simulink subsystem "PvtSubSys_VSM_ALL"  (R2020b)
settings: Solver=VariableStepAuto  StartTime=0.0  StopTime=10.0  RelTol=1e-3
values from neighbouring files (symbols this model uses):
  P_VSM_NOH_Act_Req = 0    [VSM_All.sldd]
  P_VSM_NOH_Swt_Req = 0    [VSM_All.sldd]
undefined symbols (not defined in the file or in its folder): ACC_STATE, HWA_STATE, LCK_STATE, P_VSM_ACCSOS_SW, P_VSM_AESSwtReq, P_VSM_CruiseFunUserInputMappingWays, P_VSM_ELKSwtReq, P_VSM_ESS_VehSwtReq, P_VSM_HWA_DMS_Enable, P_VSM_ICA_HandsOffSwtReq, P_VSM_IntelligentEvaSwtReq, P_VSM_ISLSwtReq, P_VSM_LCKSwtReq, P_VSM_LDWSwtReq, P_VSM_LKASwtReq, P_VSM_LSSSwtReq, P_VSM_PowerTrainConfig, P_VSM_SOSContinueTime, P_VSM_SOSSpdLimit, P_VSM_TSR_Dis_keep_SPL_Table, P_VSM_TSR_Dis_keep_SPLend, P_VSM_TSR_Dis_keep_TS_Table, P_VSM_TSR_Ena_SPLSupp_Table, P_VSM_TSR_Ena_TS_Table, P_VSM_TSR_SLIF_Speed_High, P_VSM_TSR_SLIF_Speed_Low, P_VSM_TSR_SLW_SnvtySwitch, P_VSM_TSR_SLW_Speed_Delta_disable, P_VSM_TSR_SLW_Speed_Delta_enable, P_VSM_TSR_SLW_Speed_High, P_VSM_TSR_SLW_Speed_Low, P_VSM_TSR_SLW_TrafEyeAvtiveDist, P_VSM_TSR_SLW_Warning_Time, P_VSM_TSR_SteerWheelAngle, P_VSM_TSR_SWS_speed_withDir, P_VSM_TSR_SWS_speed_woDir, P_VSM_TSRSwtReq, P_VSM_TSRWarnSwtReq, TJA_STATE, User_LC_ALCswt, User_LC_DrvConfirm, User_LC_DrvLCswt, User_LC_DrvOverride, User_LC_LeTurnNextLineReq, User_LC_RiTurnNextLineReq, User_LC_TurnMostLeLineReq, User_LC_TurnMostRiLineReq, User_LeTurnLmpOn, User_RiTurnLmpOn
libraries: simulink x51
(part 7 of 7)

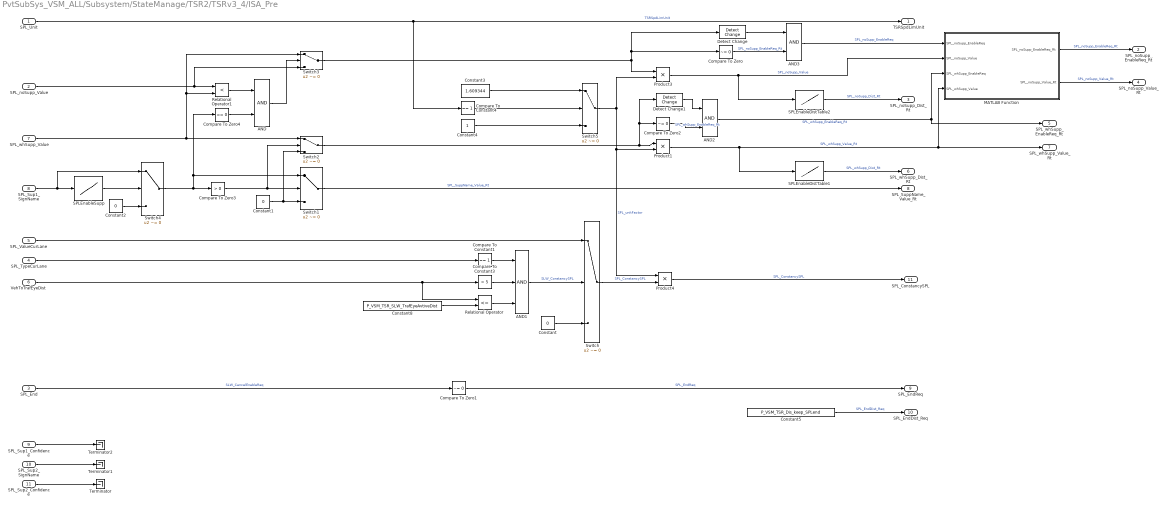
== system PvtSubSys_VSM_ALL/Subsystem/StateManage/TSR2/TSRv3_4/ISA_Pre ==
  SPL_Unit : Inport  OutDataTypeStr=uint8
  SPL_noSupp_Value : Inport  Port=2  OutDataTypeStr=uint8
  SPL_End : Inport  Port=3  OutDataTypeStr=uint8
  SPL_TypeCurLane : Inport  Port=4  OutDataTypeStr=uint8
  SPL_ValueCurLane : Inport  Port=5  OutDataTypeStr=uint8
  VehToTrafEyeDist : Inport  Port=6  OutDataTypeStr=uint16
  SPL_whSupp_Value : Inport  Port=7
  SPL_Sup1_SignName : Inport  Port=8  OutDataTypeStr=uint8
  SPL_Sup1_Confidence : Inport  Port=9  OutDataTypeStr=single
  SPL_Sup2_SignName : Inport  Port=10  OutDataTypeStr=uint8
  SPL_Sup2_Confidence : Inport  Port=11  OutDataTypeStr=single
  AND : Logic  AllPortsSameDT=off  OutDataTypeStr=boolean
  AND1 : Logic  Inputs=3  AllPortsSameDT=off  OutDataTypeStr=boolean
  AND2 : Logic  AllPortsSameDT=off  OutDataTypeStr=boolean
  AND3 : Logic  AllPortsSameDT=off  OutDataTypeStr=boolean
  Compare To Constant1 : simulink/Logic and Bit Operations/Compare To Constant  relop===  const=1  OutDataTypeStr=boolean
  Compare To Constant3 : simulink/Logic and Bit Operations/Compare To Constant  relop=>  const=5  OutDataTypeStr=boolean
  Compare To Constant4 : simulink/Logic and Bit Operations/Compare To Constant  relop===  const=1  OutDataTypeStr=boolean
  Compare To Zero : simulink/Logic and Bit Operations/Compare To Zero  relop=~=  OutDataTypeStr=boolean
  Compare To Zero1 : simulink/Logic and Bit Operations/Compare To Zero  relop=~=  OutDataTypeStr=boolean
  Compare To Zero2 : simulink/Logic and Bit Operations/Compare To Zero  relop=~=  OutDataTypeStr=boolean
  Compare To Zero3 : simulink/Logic and Bit Operations/Compare To Zero  relop=>  OutDataTypeStr=boolean
  Compare To Zero4 : simulink/Logic and Bit Operations/Compare To Zero  relop===  OutDataTypeStr=boolean
  Constant : Constant  Value=0  OutDataTypeStr=uint8
  Constant1 : Constant  Value=0  OutDataTypeStr=Inherit: Inherit via back propagation
  Constant2 : Constant  Value=0  OutDataTypeStr=Inherit: Inherit via back propagation
  Constant3 : Constant  Value=1.609344
  Constant4 : Constant
  Constant5 : Constant  Value=P_VSM_TSR_Dis_keep_SPLend  OutDataTypeStr=single
  Constant8 : Constant  Value=P_VSM_TSR_SLW_TrafEyeAvtiveDist
  Detect Change : simulink/Logic and Bit Operations/Detect Change  vinit=0  OutDataTypeStr=boolean
  Detect Change1 : simulink/Logic and Bit Operations/Detect Change  vinit=0  OutDataTypeStr=boolean
  MATLAB Function : MATLAB Function  TreatAsAtomicUnit=on
  Product1 : Product  OutDataTypeStr=uint8
  Product3 : Product  OutDataTypeStr=uint8
  Product4 : Product  OutDataTypeStr=uint8
  Relational Operator : RelationalOperator  Operator=<=  OutDataTypeStr=boolean  RndMeth=Simplest
  Relational Operator1 : RelationalOperator  Operator=<  OutDataTypeStr=boolean  RndMeth=Simplest
  SPLEnableDistTable1 : Lookup_n-D  NumberOfTableDimensions=1  BreakpointsForDimension1=[0:10:150]  BreakpointsForDimension1DataTypeStr=uint8  Table=P_VSM_TSR_Dis_keep_SPL_Table  TableDataTypeStr=Inherit: Inherit from 'Table data'  InterpMethod=Flat  ExtrapMethod=Cubic spline  InternalRulePriority=Speed  OutDataTypeStr=single  RndMeth=Simplest  InputSameDT=on
  SPLEnableDistTable2 : Lookup_n-D  NumberOfTableDimensions=1  BreakpointsForDimension1=[0:10:150]  BreakpointsForDimension1DataTypeStr=uint8  Table=P_VSM_TSR_Dis_keep_SPL_Table  TableDataTypeStr=Inherit: Inherit from 'Table data'  InterpMethod=Flat  ExtrapMethod=Cubic spline  InternalRulePriority=Speed  OutDataTypeStr=single  RndMeth=Simplest  InputSameDT=on
  SPLEnableSupp : Lookup_n-D  NumberOfTableDimensions=1  BreakpointsForDimension1=[0:1:0x16]  BreakpointsForDimension1DataTypeStr=uint8  Table=P_VSM_TSR_Ena_SPLSupp_Table  TableDataTypeStr=Inherit: Inherit from 'Table data'  InterpMethod=Flat  ExtrapMethod=Cubic spline  InternalRulePriority=Speed  OutDataTypeStr=Inherit: Inherit via back propagation  RndMeth=Simplest  InputSameDT=on
  Switch : Switch  Criteria=u2 ~= 0  OutDataTypeStr=uint8
  Switch{1..4} (4 alike) : Switch  Criteria=u2 ~= 0
  Switch5 : Switch  Criteria=u2 ~= 0  Threshold=1  OutDataTypeStr=single
  Terminator : Terminator
  Terminator1 : Terminator
  Terminator2 : Terminator
  TSRSpdLimUnit : Outport  OutDataTypeStr=uint8
  SPL_noSupp_EnableReq_Rt : Outport  Port=2  OutDataTypeStr=boolean
  SPL_noSupp_Dist_Rt : Outport  Port=3  OutDataTypeStr=single
  SPL_noSupp_Value_Rt : Outport  Port=4  OutDataTypeStr=uint8
  SPL_whSupp_EnableReq_Rt : Outport  Port=5  OutDataTypeStr=boolean
  SPL_whSupp_Dist_Rt : Outport  Port=6  OutDataTypeStr=single
  SPL_whSupp_Value_Rt : Outport  Port=7  OutDataTypeStr=uint8
  SPL_SuppName_Value_Rt : Outport  Port=8
  SPL_EndReq : Outport  Port=9  OutDataTypeStr=boolean
  SPL_EndDist_Req : Outport  Port=10  OutDataTypeStr=single
  SPL_ConstancySPL : Outport  Port=11  OutDataTypeStr=uint8
  wires:
  Compare To Zero1/1 -> SPL_EndReq/1  "SPL_EndReq"
  Switch3/1 -> Detect Change/1, Compare To Zero/1, Product3/1
  AND3/1 -> MATLAB Function/1(SPL_noSupp_EnableReq)  "SPL_noSupp_EnableReq"
  Compare To Constant3/1 -> AND1/2
  AND1/1 -> Switch/2  "SLW_ConstancySPL"
  SPL_ValueCurLane/1 -> Switch/1
  SPL_TypeCurLane/1 -> Compare To Constant1/1
  Product3/1 -> MATLAB Function/2(SPL_noSupp_Value), SPLEnableDistTable2/1  "SPL_noSupp_Value"
  Relational Operator/1 -> AND1/3
  Constant8/1 -> Relational Operator/2
  SPLEnableDistTable2/1 -> SPL_noSupp_Dist_Rt/1  "SPL_noSupp_Dist_Rt"
  Constant5/1 -> SPL_EndDist_Req/1  "SPL_EndDist_Req"
  SPL_End/1 -> Compare To Zero1/1  "SLW_CancelEnableReq"
  VehToTrafEyeDist/1 -> Relational Operator/1, Compare To Constant3/1
  Compare To Constant1/1 -> AND1/1
  Switch4/1 -> Compare To Zero4/1, Switch1/1, Compare To Zero3/1
  SPLEnableDistTable1/1 -> SPL_whSupp_Dist_Rt/1  "SPL_whSupp_Dist_Rt"
  SPL_Sup2_Confidence/1 -> Terminator/1
  SPL_Sup1_Confidence/1 -> Terminator2/1
  SPL_Sup2_SignName/1 -> Terminator1/1
  Switch2/1 -> Detect Change1/1, Compare To Zero2/1, Product1/1
  Product1/1 -> SPLEnableDistTable1/1, SPL_whSupp_Value_Rt/1, MATLAB Function/4(SPL_whSupp_Value)  "SPL_whSupp_Value_Rt"
  AND2/1 -> SPL_whSupp_EnableReq_Rt/1, MATLAB Function/3(SPL_whSupp_EnableReq)  "SPL_whSupp_EnableReq_Rt"
  Compare To Constant4/1 -> Switch5/2
  SPL_Unit/1 -> Compare To Constant4/1, TSRSpdLimUnit/1  "TSRSpdLimUnit"
  Constant3/1 -> Switch5/1
  Constant4/1 -> Switch5/3
  Switch5/1 -> Product1/2, Product4/1, Product3/2  "SPL_unitFactor"
  Constant/1 -> Switch/3
  Switch/1 -> Product4/2  "SPL_ConstancySPL"
  Product4/1 -> SPL_ConstancySPL/1  "SPL_ConstancySPL"
  Compare To Zero3/1 -> Switch2/2, Switch1/2
  SPL_whSupp_Value/1 -> Switch2/1, Switch3/1, Relational Operator1/2
  Switch1/1 -> SPL_SuppName_Value_Rt/1  "SPL_SuppName_Value_Rt"
  Constant1/1 -> Switch2/3, Switch1/3
  SPL_noSupp_Value/1 -> Switch3/3, Relational Operator1/1
  Relational Operator1/1 -> AND/1
  Compare To Zero4/1 -> AND/2
  AND/1 -> Switch3/2
  SPL_Sup1_SignName/1 -> Switch4/1, SPLEnableSupp/1
  SPLEnableSupp/1 -> Switch4/2
  Constant2/1 -> Switch4/3
  Detect Change/1 -> AND3/1
  Compare To Zero/1 -> AND3/2  "SPL_noSupp_EnableReq_Rt"
  MATLAB Function/2(SPL_noSupp_Value_Rt) -> SPL_noSupp_Value_Rt/1  "SPL_noSupp_Value_Rt"
  MATLAB Function/1(SPL_noSupp_EnableReq_Rt) -> SPL_noSupp_EnableReq_Rt/1  "SPL_noSupp_EnableReq_Rt"
  Detect Change1/1 -> AND2/1
  Compare To Zero2/1 -> AND2/2  "SPL_whSupp_EnableReq_Rt"

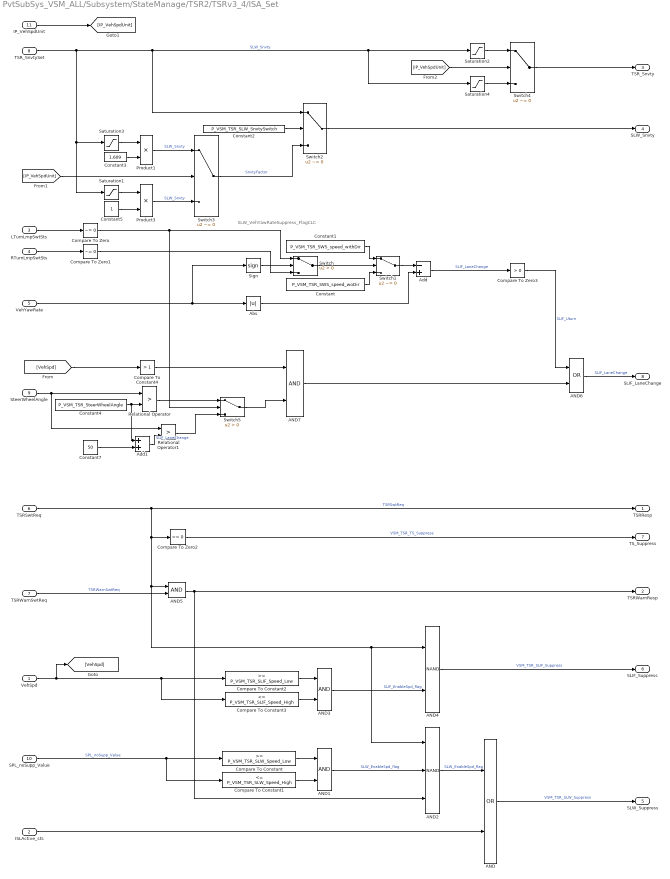
== system PvtSubSys_VSM_ALL/Subsystem/StateManage/TSR2/TSRv3_4/ISA_Set ==
  note: SLW_VehYawRateSuppress_FlagCLC
  VehSpd : Inport  OutDataTypeStr=single
  ISLActive_sts : Inport  Port=2  OutDataTypeStr=boolean
  LTurnLmpSwtSts : Inport  Port=3  OutDataTypeStr=boolean
  RTurnLmpSwtSts : Inport  Port=4  OutDataTypeStr=boolean
  VehYawRate : Inport  Port=5  OutDataTypeStr=single
  TSRSwtReq : Inport  Port=6
  TSRWarnSwtReq : Inport  Port=7
  TSR_SnvtySet : Inport  Port=8
  SteerWheelAngle : Inport  Port=9  OutDataTypeStr=single
  SPL_noSupp_Value : Inport  Port=10  OutDataTypeStr=uint8
  IP_VehSpdUnit : Inport  Port=11  OutDataTypeStr=boolean
  AND : Logic  Operator=OR  AllPortsSameDT=off  OutDataTypeStr=boolean
  AND{1,3,5,7} (4 alike) : Logic  AllPortsSameDT=off  OutDataTypeStr=boolean
  AND2 : Logic  Operator=NAND  Inputs=3  AllPortsSameDT=off  OutDataTypeStr=boolean
  AND4 : Logic  Operator=NAND  AllPortsSameDT=off  OutDataTypeStr=boolean
  AND6 : Logic  Operator=OR  AllPortsSameDT=off  OutDataTypeStr=boolean
  Abs : Abs
  Add : Sum  Inputs=-+
  Add1 : Sum
  Compare To Constant : simulink/Logic and Bit Operations/Compare To Constant  relop=>=  const=P_VSM_TSR_SLW_Speed_Low  OutDataTypeStr=boolean
  Compare To Constant1 : simulink/Logic and Bit Operations/Compare To Constant  relop=<=  const=P_VSM_TSR_SLW_Speed_High  OutDataTypeStr=boolean
  Compare To Constant2 : simulink/Logic and Bit Operations/Compare To Constant  relop=>=  const=P_VSM_TSR_SLIF_Speed_Low  OutDataTypeStr=boolean
  Compare To Constant3 : simulink/Logic and Bit Operations/Compare To Constant  relop=<=  const=P_VSM_TSR_SLIF_Speed_High  OutDataTypeStr=boolean
  Compare To Constant4 : simulink/Logic and Bit Operations/Compare To Constant  relop=>  const=1  OutDataTypeStr=boolean
  Compare To Zero : simulink/Logic and Bit Operations/Compare To Zero  relop=~=  OutDataTypeStr=boolean
  Compare To Zero1 : simulink/Logic and Bit Operations/Compare To Zero  relop=~=  OutDataTypeStr=boolean
  Compare To Zero2 : simulink/Logic and Bit Operations/Compare To Zero  relop===  OutDataTypeStr=boolean
  Compare To Zero3 : simulink/Logic and Bit Operations/Compare To Zero  relop=>  OutDataTypeStr=uint8
  Constant : Constant  Value=P_VSM_TSR_SWS_speed_woDir
  Constant1 : Constant  Value=P_VSM_TSR_SWS_speed_withDir
  Constant2 : Constant  Value=P_VSM_TSR_SLW_SnvtySwitch
  Constant3 : Constant  Value=1.609  OutDataTypeStr=single
  Constant4 : Constant  Value=P_VSM_TSR_SteerWheelAngle
  Constant5 : Constant  OutDataTypeStr=Inherit: Inherit via back propagation
  Constant7 : Constant  Value=50
  Product1 : Product  OutDataTypeStr=single
  Product3 : Product  OutDataTypeStr=single
  Relational Operator : RelationalOperator  Operator=>  OutDataTypeStr=boolean  RndMeth=Simplest
  Relational Operator1 : RelationalOperator  Operator=>  OutDataTypeStr=boolean  RndMeth=Simplest
  Saturation1 : Saturate  UpperLimit=10  LowerLimit=-10
  Saturation2 : Saturate  UpperLimit=5  LowerLimit=-5
  Saturation3 : Saturate  UpperLimit=5  LowerLimit=-5
  Saturation4 : Saturate  UpperLimit=10  LowerLimit=-10
  Sign : Signum
  Switch : Switch  Criteria=u2 > Threshold
  Switch1 : Switch  Criteria=u2 ~= 0
  Switch2 : Switch  Criteria=u2 ~= 0  OutDataTypeStr=single
  Switch3 : Switch  Criteria=u2 ~= 0  Threshold=1  OutDataTypeStr=single
  Switch4 : Switch  Criteria=u2 ~= 0  OutDataTypeStr=int8
  Switch5 : Switch  Criteria=u2 > Threshold
  TSRResp : Outport
  TSRWarnResp : Outport  Port=2
  TSR_Snvty : Outport  Port=3  OutDataTypeStr=int8
  SLW_Snvty : Outport  Port=4  OutDataTypeStr=single
  SLW_Suppress : Outport  Port=5
  SLIF_Suppress : Outport  Port=6
  TS_Suppress : Outport  Port=7
  SLIF_LaneChange : Outport  Port=8  OutDataTypeStr=boolean
  wires:
  AND4/1 -> SLIF_Suppress/1  "VSM_TSR_SLIF_Suppress"
  Abs/1 -> Add/2
  VehYawRate/1 -> Abs/1, Sign/1
  Sign/1 -> Switch/2
  Compare To Zero/1 -> Switch/1, Switch5/2
  RTurnLmpSwtSts/1 -> Compare To Zero1/1
  Switch1/1 -> Add/1
  Compare To Zero1/1 -> Switch/3
  Constant/1 -> Switch1/3
  Switch/1 -> Switch1/2
  Constant1/1 -> Switch1/1
  LTurnLmpSwtSts/1 -> Compare To Zero/1
  Add/1 -> Compare To Zero3/1  "SLIF_LaneChange"
  AND/1 -> SLW_Suppress/1  "VSM_TSR_SLW_Suppress"
  ISLActive_sts/1 -> AND/2
  Compare To Constant1/1 -> AND1/2
  Compare To Constant/1 -> AND1/1
  AND1/1 -> AND2/2  "SLW_EnableSpd_flag"
  AND5/1 -> AND2/3, TSRWarnResp/1
  AND2/1 -> AND/1  "SLW_EnableSpd_flag"
  Compare To Constant2/1 -> AND3/1
  AND3/1 -> AND4/2  "SLIF_EnableSpd_flag"
  Compare To Constant3/1 -> AND3/2
  VehSpd/1 -> [VehSpd], Compare To Constant3/1, Compare To Constant2/1
  TSRSwtReq/1 -> Compare To Zero2/1, AND2/1, AND4/1, AND5/1, TSRResp/1  "TSRSwtReq"
  TSRWarnSwtReq/1 -> AND5/2  "TSRWarnSwtReq"
  Compare To Zero2/1 -> TS_Suppress/1  "VSM_TSR_TS_Suppress"
  Compare To Zero3/1 -> AND6/1  "SLIF_Uturn"
  Constant2/1 -> Switch2/2
  Switch2/1 -> SLW_Snvty/1
  SteerWheelAngle/1 -> Relational Operator1/1, Relational Operator/1
  Constant4/1 -> Add1/1, Relational Operator/2
  Switch5/1 -> AND7/2
  AND6/1 -> SLIF_LaneChange/1  "SLIF_LaneChange"
  [VehSpd] -> Compare To Constant4/1
  Compare To Constant4/1 -> AND7/1
  AND7/1 -> AND6/2
  SPL_noSupp_Value/1 -> Compare To Constant1/1, Compare To Constant/1  "SPL_noSupp_Value"
  Switch3/1 -> Switch2/3  "SnvtyFactor"
  [IP_VehSpdUnit] -> Switch3/2
  Constant5/1 -> Product3/2
  TSR_SnvtySet/1 -> Saturation1/1, Saturation3/1, Switch2/1, Saturation4/1, Saturation2/1  "SLW_Snvty"
  Constant3/1 -> Product1/2
  Product1/1 -> Switch3/1  "SLW_Snvty"
  Product3/1 -> Switch3/3  "SLW_Snvty"
  Saturation3/1 -> Product1/1
  Saturation1/1 -> Product3/1
  Switch4/1 -> TSR_Snvty/1
  IP_VehSpdUnit/1 -> [IP_VehSpdUnit]
  [IP_VehSpdUnit] -> Switch4/2
  Saturation2/1 -> Switch4/1
  Saturation4/1 -> Switch4/3
  Relational Operator/1 -> Switch5/1
  Constant7/1 -> Add1/2
  Add1/1 -> Relational Operator1/2  "SLIF_LaneChange"
  Relational Operator1/1 -> Switch5/3

== system PvtSubSys_VSM_ALL/Subsystem/StateManage/TSR2/TSRv3_4/ISAnoSupp ==
  SLW_Snvty : Inport  OutDataTypeStr=single
  SLIF_VehSpdValue : Inport  Port=2  OutDataTypeStr=single
  SLIF_LaneChange : Inport  Port=3  OutDataTypeStr=boolean
  SLIF_Suppress : Inport  Port=4  OutDataTypeStr=boolean
  SLW_Suppress : Inport  Port=5
  SPL_noSupp_EnableReq : Inport  Port=6  OutDataTypeStr=boolean
  SPL_noSupp_Dist_Req : Inport  Port=7  OutDataTypeStr=single
  SPL_noSupp_Value_Req : Inport  Port=8  OutDataTypeStr=uint8
  SPL_End_Req : Inport  Port=9  OutDataTypeStr=boolean
  SPL_EndDist_Req : Inport  Port=10  OutDataTypeStr=single
  SPL_Constancy_Req : Inport  Port=11  OutDataTypeStr=uint8
  Chart1 : Stateflow chart  TreatAsAtomicUnit=on
  Constant : Constant  Value=0  OutDataTypeStr=Inherit: Inherit via back propagation
  Constant1 : Constant  Value=P_VSM_TSR_SLW_Speed_Delta_enable
  Constant13 : Constant  Value=P_VSM_TSR_SLW_Warning_Time
  Constant2 : Constant  Value=P_VSM_TSR_SLW_SnvtySwitch
  Constant3 : Constant  Value=P_VSM_TSR_SLW_Speed_Delta_disable
  Ground : Ground
  Switch{,1..3} (4 alike) : Switch  Criteria=u2 ~= 0
  Switch4 : Switch  Criteria=u2 ~= 0  OutDataTypeStr=single
  Terminator : Terminator
  Terminator1 : Terminator
  Unit Delay : UnitDelay  SampleTime=-1  HasFrameUpgradeWarning=on
  TSRSpdLimWarn : Outport
  TSRSpdLimCfdc : Outport  Port=2  OutDataTypeStr=uint8
  TSRSpdLim : Outport  Port=3
  TSRSpdLimSts : Outport  Port=4
  SLW_Enable : Outport  Port=5
  SLW_SpdLimValue : Outport  Port=6  OutDataTypeStr=uint8
  SPL_noSupp_Dist_Remain : Outport  Port=7  OutDataTypeStr=single
  SPLnoSuppDistKeep : Outport  Port=8
  SPL_noSupp_Value_Remain : Outport  Port=9
  wires:
  SLIF_Suppress/1 -> Switch/2, Switch1/2, Switch2/2  "SLIF_Suppress"
  SLIF_VehSpdValue/1 -> Chart1/1(SLIF_VehSpdValue)
  Chart1/4(TSRSpdLimWarn) -> SLW_Enable/1, Switch3/3  "SLW_Enable"
  Chart1/8(SLIF_SpdLimValue) -> Unit Delay/1, SPL_noSupp_Value_Remain/1  "SPL_noSupp_Value_Remain"
  Chart1/3(SLIF_SpdLimCoded) -> Switch2/3
  Chart1/6(SLIF_EnableDist) -> SPLnoSuppDistKeep/1  "SPLdistKeep"
  Chart1/7(SLIF_RemainDist) -> SPL_noSupp_Dist_Remain/1  "SPL_noSupp_Dist_Remain"
  Chart1/1(TSRSpdLimSts) -> Switch/3
  Chart1/9(SLW_SpdLimValue) -> SLW_SpdLimValue/1  "SLW_SpdLimValue"
  Chart1/2(TSRSpdLimCfdc) -> Switch1/3
  Switch/1 -> TSRSpdLimSts/1  "TSRSpdLimSts"
  Switch1/1 -> TSRSpdLimCfdc/1  "TSRSpdLimCfdc"
  Switch2/1 -> TSRSpdLim/1  "TSRSpdLim"
  Switch3/1 -> TSRSpdLimWarn/1  "TSRSpdLimWarn"
  SLW_Suppress/1 -> Switch3/2
  Constant/1 -> Switch3/1, Switch2/1, Switch1/1, Switch/1
  Constant1/1 -> Chart1/10(APV_SLW_Speed_Delta_enable)
  Constant3/1 -> Chart1/11(APV_SLW_Speed_Delta_disable)
  Constant13/1 -> Chart1/12(APV_SLW_Warning_Time)
  SPL_noSupp_EnableReq/1 -> Chart1/3(SLIF_EnableReq)  "VSM_TSR_SPL_noSupp_EnableReq"
  SPL_noSupp_Dist_Req/1 -> Chart1/4(SLIF_EnableDistReq)  "VSM_TSR_SPL_noSupp_Dist_Req"
  SPL_noSupp_Value_Req/1 -> Chart1/5(SLIF_SpdLimValueReq)  "VSM_TSR_SPL_noSupp_Value_Req"
  SPL_Constancy_Req/1 -> Chart1/6(SLIF_ConstancySPL)  "VSM_TSR_SPL_Constancy_Req"
  SPL_End_Req/1 -> Chart1/7(SLIF_End_Req)  "VSM_TSR_SPL_End_Req"
  SPL_EndDist_Req/1 -> Chart1/8(SLIF_EndDist_Req)  "VSM_TSR_SPL_EndDist_Req"
  SLIF_LaneChange/1 -> Chart1/9(SLIF_Disable)
  Ground/1 -> Chart1/13(SPL_SuppName_Value_Req)
  Chart1/10(SPL_SuppName) -> Terminator/1
  Constant2/1 -> Switch4/2
  SLW_Snvty/1 -> Switch4/3  "SLW_Snvty"
  Switch4/1 -> Chart1/2(SLW_Snvty)
  Unit Delay/1 -> Switch4/1
  Chart1/5(SLIF_Enable) -> Terminator1/1  "SLW_Enable"

== system PvtSubSys_VSM_ALL/Subsystem/StateManage/TSR2/TSRv3_4/ISAwhSupp ==
  SLW_Snvty : Inport  OutDataTypeStr=single
  SLIF_VehSpdValue : Inport  Port=2
  SLIF_LaneChange : Inport  Port=3  OutDataTypeStr=boolean
  SLIF_Suppress : Inport  Port=4  OutDataTypeStr=boolean
  SLW_Suppress : Inport  Port=5
  SPL_whSupp_EnableReq : Inport  Port=6  OutDataTypeStr=boolean
  SPL_whSupp_Dist_Req : Inport  Port=7  OutDataTypeStr=single
  SPL_whSupp_Value_Req : Inport  Port=8  OutDataTypeStr=uint8
  SPL_SuppName_Value_Req : Inport  Port=9  OutDataTypeStr=uint8
  SPL_End_Req : Inport  Port=10  OutDataTypeStr=boolean
  SPL_EndDist_Req : Inport  Port=11  OutDataTypeStr=single
  SPL_Constancy_Req : Inport  Port=12  OutDataTypeStr=uint8
  Chart1 : Stateflow chart  TreatAsAtomicUnit=on
  Constant : Constant  Value=0  OutDataTypeStr=Inherit: Inherit via back propagation
  Constant1 : Constant  Value=P_VSM_TSR_SLW_Speed_Delta_enable
  Constant13 : Constant  Value=P_VSM_TSR_SLW_Warning_Time
  Constant2 : Constant  Value=P_VSM_TSR_SLW_SnvtySwitch
  Constant3 : Constant  Value=P_VSM_TSR_SLW_Speed_Delta_disable
  Switch2 : Switch  Criteria=u2 ~= 0
  Switch3 : Switch  Criteria=u2 ~= 0
  Switch4 : Switch  Criteria=u2 ~= 0  OutDataTypeStr=single
  Terminator{,1,3..4} (4 alike) : Terminator
  Unit Delay : UnitDelay  SampleTime=-1  HasFrameUpgradeWarning=on
  TSRConSpdLimWarn : Outport
  TSRConSpdLim : Outport  Port=2
  SPL_whSupp_Dist_Remain : Outport  Port=3  OutDataTypeStr=single
  SPL_whSupp_Value_Remain : Outport  Port=4  OutDataTypeStr=uint8
  SPL_SuppName_Value_Remain : Outport  Port=5  OutDataTypeStr=uint8
  SPLwhSuppDistKeep : Outport  Port=6  OutDataTypeStr=single
  wires:
  Constant/1 -> Switch2/1, Switch3/1
  Chart1/2(TSRSpdLimCfdc) -> Terminator1/1
  Chart1/1(TSRSpdLimSts) -> Terminator/1
  SLW_Suppress/1 -> Switch3/2
  Chart1/4(TSRSpdLimWarn) -> Switch3/3
  Switch2/1 -> TSRConSpdLim/1  "TSRConSpdLim"
  Chart1/3(SLIF_SpdLimCoded) -> Switch2/3
  SPL_EndDist_Req/1 -> Chart1/8(SLIF_EndDist_Req)
  Chart1/6(SLIF_EnableDist) -> SPLwhSuppDistKeep/1  "SPLwhSuppDistKeep"
  Switch3/1 -> TSRConSpdLimWarn/1  "TSRConSpdLimWarn"
  Chart1/5(SLIF_Enable) -> Terminator4/1
  SPL_End_Req/1 -> Chart1/7(SLIF_End_Req)
  SPL_Constancy_Req/1 -> Chart1/6(SLIF_ConstancySPL)
  SLIF_Suppress/1 -> Switch2/2  "SLIF_Suppress"
  SPL_whSupp_EnableReq/1 -> Chart1/3(SLIF_EnableReq)  "VSM_TSR_SPL_whSupp_EnableReq"
  Chart1/7(SLIF_RemainDist) -> SPL_whSupp_Dist_Remain/1  "SPL_whSupp_Dist_Remain"
  SPL_whSupp_Value_Req/1 -> Chart1/5(SLIF_SpdLimValueReq)  "VSM_TSR_SPL_whSupp_Value_Req"
  SLIF_VehSpdValue/1 -> Chart1/1(SLIF_VehSpdValue)
  SPL_whSupp_Dist_Req/1 -> Chart1/4(SLIF_EnableDistReq)  "VSM_TSR_SPL_whSupp_Dist_Req"
  Chart1/10(SPL_SuppName) -> SPL_SuppName_Value_Remain/1  "SPL_SuppName_Value_Remain"
  SLIF_LaneChange/1 -> Chart1/9(SLIF_Disable)
  Chart1/9(SLW_SpdLimValue) -> Terminator3/1
  SPL_SuppName_Value_Req/1 -> Chart1/13(SPL_SuppName_Value_Req)
  Constant1/1 -> Chart1/10(APV_SLW_Speed_Delta_enable)
  Constant3/1 -> Chart1/11(APV_SLW_Speed_Delta_disable)
  Constant13/1 -> Chart1/12(APV_SLW_Warning_Time)
  Constant2/1 -> Switch4/2
  Chart1/8(SLIF_SpdLimValue) -> Unit Delay/1, SPL_whSupp_Value_Remain/1  "SPL_whSupp_Value_Remain"
  Switch4/1 -> Chart1/2(SLW_Snvty)
  SLW_Snvty/1 -> Switch4/3  "SLW_Snvty"
  Unit Delay/1 -> Switch4/1

== system PvtSubSys_VSM_ALL/Subsystem/StateManage/TSR2/TSRv3_4/TSIF ==
  SPL_SuppName : Inport
  TSD_VehSpdValue : Inport  Port=2
  TSIF_Suppress : Inport  Port=3
  TSIF_EnableReq : Inport  Port=4  OutDataTypeStr=boolean
  TSIF_EnableDistReq : Inport  Port=5  OutDataTypeStr=single
  TSD_TSValueReq : Inport  Port=6  OutDataTypeStr=uint8
  Chart2 : Stateflow chart  TreatAsAtomicUnit=on
  Constant : Constant  Value=0  OutDataTypeStr=Inherit: Inherit via back propagation
  Switch : Switch  Criteria=u2 > Threshold
  TSRTrfcSignVal : Outport
  TSRTrfcSignValCfdc : Outport  Port=2
  TS_SignName_Value_Remain : Outport  Port=3
  TS_SignName_Dist_Remain : Outport  Port=4
  TSDistKeep : Outport  Port=5
  wires:
  TSIF_EnableDistReq/1 -> Chart2/3(TSIF_EnableDistReq)
  TSIF_EnableReq/1 -> Chart2/2(TSIF_EnableReq)
  TSD_TSValueReq/1 -> Chart2/4(TSIF_SignName_Req)
  TSD_VehSpdValue/1 -> Chart2/1(TSIF_VehSpdValue)
  TSIF_Suppress/1 -> Switch/2
  SPL_SuppName/1 -> Chart2/5(TSIF_ConstancyTS)
  Chart2/3(TSIF_TSConfidence) -> TSRTrfcSignValCfdc/1  "TSRTrfcSignValCfdc"
  Chart2/5(TSIF_RemainDist) -> TS_SignName_Dist_Remain/1  "TS_SignName_Dist_Remain"
  Chart2/4(TSIF_EnableDist) -> TSDistKeep/1  "TSDistKeep"
  Chart2/2(TSIF_SignName_Rm) -> TS_SignName_Value_Remain/1  "TS_SignName_Value_Remain"
  Chart2/1(TSIF_SignName) -> Switch/3
  Switch/1 -> TSRTrfcSignVal/1  "TSRTrfcSignVal"
  Constant/1 -> Switch/1

== system PvtSubSys_VSM_ALL/Subsystem/StateManage/TSR2/TSRv3_4/TSIF_Pre ==
  TSR_Sign_Name : Inport
  TS_Confidence : Inport  Port=2  OutDataTypeStr=single
  1-D Lookup Table : Lookup_n-D  NumberOfTableDimensions=1  BreakpointsForDimension1=[0:47]  BreakpointsForDimension1DataTypeStr=uint8  Table=P_VSM_TSR_Dis_keep_TS_Table  TableDataTypeStr=Inherit: Inherit from 'Table data'  InterpMethod=Nearest  InternalRulePriority=Speed  OutDataTypeStr=single  RndMeth=Simplest  InputSameDT=on
  1-D Lookup Table2 : Lookup_n-D  NumberOfTableDimensions=1  BreakpointsForDimension1=[0:47]  Table=P_VSM_TSR_Ena_TS_Table  TableDataTypeStr=Inherit: Inherit from 'Table data'  InterpMethod=Nearest  InternalRulePriority=Speed  RndMeth=Simplest  InputSameDT=on
  AND : Logic  AllPortsSameDT=off  OutDataTypeStr=boolean
  Compare To Zero : simulink/Logic and Bit Operations/Compare To Zero  relop=~=  OutDataTypeStr=boolean
  Terminator : Terminator
  TS_SignName_EnableReq_Rt : Outport
  TS_SignName_Dist_Rt : Outport  Port=2  OutDataTypeStr=single
  TS_SignName_Value_Rt : Outport  Port=3
  wires:
  TSR_Sign_Name/1 -> 1-D Lookup Table/1, TS_SignName_Value_Rt/1, 1-D Lookup Table2/1, Compare To Zero/1  "TS_SignName_Value_Rt"
  1-D Lookup Table/1 -> TS_SignName_Dist_Rt/1  "TSD_EnableDistReq"
  Compare To Zero/1 -> AND/2
  1-D Lookup Table2/1 -> AND/1
  AND/1 -> TS_SignName_EnableReq_Rt/1  "TSD_EnableReq"
  TS_Confidence/1 -> Terminator/1

== matlab function PvtSubSys_VSM_ALL/Subsystem/StateManage/TSR2/TSRv3_4/ISA_Pre/MATLAB Function ==
  data: SPL_noSupp_EnableReq input; SPL_noSupp_EnableReq_Rt output; SPL_noSupp_Value input; SPL_whSupp_EnableReq input; SPL_whSupp_Value input; SPL_noSupp_Value_Rt output
function [SPL_noSupp_EnableReq_Rt, SPL_noSupp_Value_Rt]= fcn(SPL_noSupp_EnableReq, SPL_noSupp_Value,SPL_whSupp_EnableReq,SPL_whSupp_Value)

if SPL_whSupp_EnableReq>0
    SPL_noSupp_EnableReq_Rt=SPL_whSupp_EnableReq;
    SPL_noSupp_Value_Rt=SPL_whSupp_Value;
else
    SPL_noSupp_EnableReq_Rt=SPL_noSupp_EnableReq;
    SPL_noSupp_Value_Rt=SPL_noSupp_Value;
end
end

== stateflow chart PvtSubSys_VSM_ALL/Subsystem/StateManage/TSR2/TSRv3_4/ISAnoSupp/Chart1 ==
  state ConstancySPL
    SLIF_Enable=true;
    SLIF_SpdLimValue=SLIF_ConstancySPL;
    SLIF_SpdLimCoded=SLIF_SpdLimValue/5;
    SLIF_EnableDist=single(0);
    TSRSpdLimCfdc=uint8(2);
    SLW_SpdLimValue = SLIF_SpdLimValue + uint8(SLW_Snvty);
    SLW_SpdEnterThresh= SLW_SpdLimValue + APV_SLW_Speed_Delta_enable;
    SLW_SpdExitThresh = SLW_SpdLimValue - APV_SLW_Speed_Delta_disable;
    du:
    SLW_Vehicle_Speed=SLIF_VehSpdValue*1.03+1.3-SLW_Snvty;
    state No_Warning
      du:TSRSpdLimWarn=false;
    state Warning
      en:i=0;
      du:i=i+1;
      TSRSpdLimWarn=true;
    state Enouth_Warning
      du:TSRSpdLimWarn=false;
    ConstancySPL.Warning -> ConstancySPL.No_Warning [order 1] : [SLW_Vehicle_Speed<=SLW_SpdExitThresh]
    (default) -> ConstancySPL.No_Warning
    ConstancySPL.No_Warning -> ConstancySPL.Warning : [SLW_Vehicle_Speed>SLW_SpdEnterThresh]
    ConstancySPL.Enouth_Warning -> ConstancySPL.No_Warning : [SLW_Vehicle_Speed<=SLW_SpdExitThresh]
    ConstancySPL.Warning -> ConstancySPL.Enouth_Warning [order 2] : [(i>(APV_SLW_Warning_Time/0.02))]
  state Disable
    SLIF_Enable=false;
    SLIF_SpdLimValue=uint8(0);
    SLIF_EnableDist=single(0);
    TSRSpdLimSts=uint8(0);
    TSRSpdLimCfdc=uint8(0);
    SLIF_SpdLimCoded=uint8(0);
    SPL_SuppName=uint8(0);
    TSRSpdLimWarn=false;
  state SPLend
    en:
    SLIF_SPLendTotalDist=single(0);
    SLIF_RemainDist=single(0);
    SLIF_EndDist=SLIF_EndDist_Req;
    TSRSpdLimWarn=false;
    SLIF_SpdLimValue=uint8(0);
    SLIF_SpdLimCoded=uint8(0);
    TSRSpdLimSts=uint8(2);
    du:
    SLIF_SPLendTotalDist=SLIF_SPLendTotalDist+SLIF_VehSpdValue*0.02/3.6;
    ex:
    SLIF_SPLendTotalDist=single(0);
  state SPL
    state Ready
      SLIF_SpdLimValue=SLIF_SpdLimValueReq;
      SLIF_EnableDist=SLIF_EnableDistReq;
      SLIF_SPLTotalDist=0;
      SPL_SuppName=SPL_SuppName_Value_Req;
    state Enable
      en:
      TSRSpdLimSts=uint8(1);
      TSRSpdLimCfdc=uint8(2);
      SLIF_SpdLimCoded=SLIF_SpdLimValue/5;
      SLIF_Enable=true;
      SLW_SpdLimValue = SLIF_SpdLimValue + uint8(SLW_Snvty);
      SLW_SpdEnterThresh= SLW_SpdLimValue + APV_SLW_Speed_Delta_enable;
      SLW_SpdExitThresh = SLW_SpdLimValue - APV_SLW_Speed_Delta_disable;
      du:
      SLIF_SPLTotalDist=SLIF_SPLTotalDist+SLIF_VehSpdValue*0.02/3.6;
      SLIF_RemainDist=SLIF_EnableDist-SLIF_SPLTotalDist;
      SLW_Vehicle_Speed=SLIF_VehSpdValue*1.03+1.3;
      state No_Warning
        du:TSRSpdLimWarn=false;
      state Warning
        en:i=0;
        du:i=i+1;
        TSRSpdLimWarn=true;
      state Enouth_Warning
        du:TSRSpdLimWarn=false;
      SPL.Enable.Warning -> SPL.Enable.No_Warning [order 1] : [SLW_Vehicle_Speed<=SLW_SpdExitThresh]
      (default) -> SPL.Enable.No_Warning
      SPL.Enable.No_Warning -> SPL.Enable.Warning : [SLW_Vehicle_Speed>SLW_SpdEnterThresh]
      SPL.Enable.Enouth_Warning -> SPL.Enable.No_Warning : [SLW_Vehicle_Speed<=SLW_SpdExitThresh]
      SPL.Enable.Warning -> SPL.Enable.Enouth_Warning [order 2] : [(i>(uint16(APV_SLW_Warning_Time)/0.02))]
    (default) -> Ready
    Enable -> Ready : [SLIF_EnableReq]
    Ready -> Enable : [~SLIF_EnableReq]
  ConstancySPL -> Disable [order 1] : [(SLIF_ConstancySPL==0)...
      | &&(~SLIF_EnableReq)]
  Disable -> ConstancySPL [order 2] : [SLIF_ConstancySPL~=0]
  ConstancySPL -> SPLend [order 3] : [SLIF_End_Req]
  ConstancySPL -> SPL [order 2] : [SLIF_EnableReq]
  (default) -> Disable
  SPLend -> Disable [order 2] : [SLIF_SPLendTotalDist>SLIF_EnableDist]
  SPL -> Disable [order 1] : [SLIF_SPLTotalDist>=SLIF_EnableDist...
      | ||SLIF_Disable]
  Disable -> SPL [order 1] : [SLIF_EnableReq]
  SPL -> SPLend [order 2] : [SLIF_End_Req]
  SPLend -> SPL [order 1] : [SLIF_EnableReq]
  data: TSRSpdLimSts output; TSRSpdLimCfdc output; SLIF_SpdLimCoded output uint8; TSRSpdLimWarn output; SLIF_Enable output boolean; SLIF_VehSpdValue input; SLW_Snvty input; SLIF_EnableReq input; SLIF_EnableDistReq input single; SLIF_EnableDist output single; SLIF_RemainDist output single; SLIF_SpdLimValue output uint8; SLIF_SpdLimValueReq input uint8; SLIF_ConstancySPL input uint8; i local; SLW_SpdEnterThresh local; SLW_SpdExitThresh local; SLW_Vehicle_Speed local; SLW_SpdLimValue output; SLIF_SPLTotalDist local single; SLIF_End_Req input boolean; SLIF_EndDist_Req input single; SLIF_SPLendTotalDist local single; SLIF_EndDist local single; SLIF_Disable input; APV_SLW_Speed_Delta_enable input; APV_SLW_Speed_Delta_disable input; APV_SLW_Warning_Time input; SLIF_SpdLimValue_Hold local uint8; SPL_SuppName_Value_Req input uint8; SPL_SuppName output uint8

== stateflow chart PvtSubSys_VSM_ALL/Subsystem/StateManage/TSR2/TSRv3_4/ISAwhSupp/Chart1 ==
  state ConstancySPL
    SLIF_Enable=true;
    SLIF_SpdLimValue=SLIF_ConstancySPL;
    SLIF_SpdLimCoded=SLIF_SpdLimValue/5;
    SLIF_EnableDist=single(0);
    TSRSpdLimCfdc=uint8(2);
    SLW_SpdLimValue = SLIF_SpdLimValue + uint8(SLW_Snvty);
    SLW_SpdEnterThresh= SLW_SpdLimValue + APV_SLW_Speed_Delta_enable;
    SLW_SpdExitThresh = SLW_SpdLimValue - APV_SLW_Speed_Delta_disable;
    du:
    SLW_Vehicle_Speed=SLIF_VehSpdValue*1.03+1.3-SLW_Snvty;
    state No_Warning
      du:TSRSpdLimWarn=false;
    state Warning
      en:i=0;
      du:i=i+1;
      TSRSpdLimWarn=true;
    state Enouth_Warning
      du:TSRSpdLimWarn=false;
    ConstancySPL.Warning -> ConstancySPL.No_Warning [order 1] : [SLW_Vehicle_Speed<=SLW_SpdExitThresh]
    (default) -> ConstancySPL.No_Warning
    ConstancySPL.No_Warning -> ConstancySPL.Warning : [SLW_Vehicle_Speed>SLW_SpdEnterThresh]
    ConstancySPL.Enouth_Warning -> ConstancySPL.No_Warning : [SLW_Vehicle_Speed<=SLW_SpdExitThresh]
    ConstancySPL.Warning -> ConstancySPL.Enouth_Warning [order 2] : [(i>(APV_SLW_Warning_Time/0.02))]
  state SPLend
    en:
    SLIF_SPLendTotalDist=single(0);
    SLIF_RemainDist=single(0);
    SLIF_EndDist=SLIF_EndDist_Req;
    TSRSpdLimWarn=false;
    SLIF_SpdLimValue=uint8(0);
    SLIF_SpdLimCoded=uint8(0);
    TSRSpdLimSts=uint8(2);
    du:
    SLIF_SPLendTotalDist=SLIF_SPLendTotalDist+SLIF_VehSpdValue*0.02/3.6;
    ex:
    SLIF_SPLendTotalDist=single(0);
  state Disable
    SLIF_Enable=false;
    SLIF_SpdLimValue=uint8(0);
    SLIF_EnableDist=single(0);
    TSRSpdLimSts=uint8(0);
    TSRSpdLimCfdc=uint8(0);
    SLIF_SpdLimCoded=uint8(0);
    SPL_SuppName=uint8(0);
    TSRSpdLimWarn=false;
  state SPL
    state Ready
      SLIF_SpdLimValue=SLIF_SpdLimValueReq;
      SLIF_EnableDist=SLIF_EnableDistReq;
      SLIF_SPLTotalDist=0;
      SPL_SuppName=SPL_SuppName_Value_Req;
    state Enable
      en:
      TSRSpdLimSts=uint8(1);
      TSRSpdLimCfdc=uint8(2);
      SLIF_SpdLimCoded=SLIF_SpdLimValue/5;
      SLIF_Enable=true;
      SLW_SpdLimValue = SLIF_SpdLimValue + uint8(SLW_Snvty);
      SLW_SpdEnterThresh= SLW_SpdLimValue + APV_SLW_Speed_Delta_enable;
      SLW_SpdExitThresh = SLW_SpdLimValue - APV_SLW_Speed_Delta_disable;
      du:
      SLIF_SPLTotalDist=SLIF_SPLTotalDist+SLIF_VehSpdValue*0.02/3.6;
      SLIF_RemainDist=SLIF_EnableDist-SLIF_SPLTotalDist;
      SLW_Vehicle_Speed=SLIF_VehSpdValue*1.03+1.3;
      state No_Warning
        du:TSRSpdLimWarn=false;
      state Warning
        en:i=0;
        du:i=i+1;
        TSRSpdLimWarn=true;
      state Enouth_Warning
        du:TSRSpdLimWarn=false;
      SPL.Enable.Warning -> SPL.Enable.No_Warning [order 1] : [SLW_Vehicle_Speed<=SLW_SpdExitThresh]
      (default) -> SPL.Enable.No_Warning
      SPL.Enable.No_Warning -> SPL.Enable.Warning : [SLW_Vehicle_Speed>SLW_SpdEnterThresh]
      SPL.Enable.Enouth_Warning -> SPL.Enable.No_Warning : [SLW_Vehicle_Speed<=SLW_SpdExitThresh]
      SPL.Enable.Warning -> SPL.Enable.Enouth_Warning [order 2] : [(i>(uint16(APV_SLW_Warning_Time)/0.02))]
    (default) -> Ready
    Enable -> Ready : [SLIF_EnableReq]
    Ready -> Enable : [~SLIF_EnableReq]
  ConstancySPL -> Disable [order 1] : [(SLIF_ConstancySPL==0)...
      | &&(~SLIF_EnableReq)]
  Disable -> ConstancySPL [order 2] : [SLIF_ConstancySPL~=0]
  ConstancySPL -> SPLend [order 3] : [SLIF_End_Req]
  ConstancySPL -> SPL [order 2] : [SLIF_EnableReq]
  (default) -> Disable
  SPLend -> Disable [order 2] : [SLIF_SPLendTotalDist>SLIF_EnableDist]
  SPL -> Disable [order 1] : [SLIF_SPLTotalDist>=SLIF_EnableDist...
      | ||SLIF_Disable]
  Disable -> SPL [order 1] : [SLIF_EnableReq]
  SPL -> SPLend [order 2] : [SLIF_End_Req]
  SPLend -> SPL [order 1] : [SLIF_EnableReq]
  data: TSRSpdLimSts output; TSRSpdLimCfdc output; SLIF_SpdLimCoded output uint8; TSRSpdLimWarn output; SLIF_Enable output boolean; SLIF_VehSpdValue input; SLW_Snvty input; SLIF_EnableReq input; SLIF_EnableDistReq input single; SLIF_EnableDist output single; SLIF_RemainDist output single; SLIF_SpdLimValue output uint8; SLIF_SpdLimValueReq input uint8; SLIF_ConstancySPL input uint8; i local; SLW_SpdEnterThresh local; SLW_SpdExitThresh local; SLW_Vehicle_Speed local; SLW_SpdLimValue output; SLIF_SPLTotalDist local single; SLIF_End_Req input boolean; SLIF_EndDist_Req input single; SLIF_SPLendTotalDist local single; SLIF_EndDist local single; SLIF_Disable input; APV_SLW_Speed_Delta_enable input; APV_SLW_Speed_Delta_disable input; APV_SLW_Warning_Time input; SLIF_SpdLimValue_Hold local uint8; SPL_SuppName_Value_Req input uint8; SPL_SuppName output uint8

== stateflow chart PvtSubSys_VSM_ALL/Subsystem/StateManage/TSR2/TSRv3_4/TSIF/Chart2 ==
  state ConstancyTS
    TSIF_SignName=TSIF_ConstancyTS+0x2f;
    TSIF_SignName_Rm=uint8(0);
    TSIF_EnableDist=single(0);
    TSIF_TSConfidence=uint8(2);
    TSIF_RemainDist=single(0);
  state Disable
    TSIF_SignName=uint8(0);
    TSIF_SignName_Rm=uint8(0);
    TSIF_EnableDist=single(0);
    TSIF_TSConfidence=uint8(0);
  state SPL
    state Ready
      TSIF_SignName=TSIF_SignName_Req;
      TSIF_SignName_Rm=TSIF_SignName_Req;
      TSIF_EnableDist=TSIF_EnableDistReq;
      TSIF_TSTotalDist=0;
    state Enable
      du:
      TSIF_TSTotalDist=TSIF_TSTotalDist+TSIF_VehSpdValue*0.02/3.6;
      TSIF_RemainDist=TSIF_EnableDist-TSIF_TSTotalDist;
      TSIF_TSConfidence=uint8(2);
    (default) -> Ready
    Enable -> Ready : [TSIF_EnableReq]
    Ready -> Enable : [~TSIF_EnableReq]
  ConstancyTS -> Disable : [TSIF_ConstancyTS==0]
  Disable -> ConstancyTS [order 2] : [TSIF_ConstancyTS~=0]
  SPL -> ConstancyTS [order 2] : [TSIF_ConstancyTS~=0]
  (default) -> Disable
  SPL -> Disable [order 1] : [TSIF_TSTotalDist>=TSIF_EnableDist]
  Disable -> SPL [order 1] : [TSIF_EnableReq]
  data: TSIF_SignName output uint8 size=1; TSIF_SignName_Rm output uint8 size=1; TSIF_TSConfidence output uint8 size=1; TSIF_VehSpdValue input single size=1; TSIF_EnableReq input boolean size=1; TSIF_EnableDistReq input single size=1; TSIF_EnableDist output single size=1; TSIF_RemainDist output single size=1; TSIF_SignName_Req input uint8 size=1; TSIF_ConstancyTS input uint8 size=1; TSIF_TSTotalDist local single size=1

== stateflow chart PvtSubSys_VSM_ALL/Subsystem/StateManage/TSR2/TSRv3_4/TSRSM ==
  state Start
  state INIT
    SPL_noSupp_Value_Req=SPL_noSupp_Value_Init;
    SPL_noSupp_Dist_Req=SPL_noSupp_Dist_Init;
    SPL_whSupp_Dist_Req=SPL_whSupp_Dist_Init;
    SPL_whSupp_Value_Req=SPL_whSupp_Value_Init;
    SPL_SuppName_Value_Req=SPL_SuppName_Value_Init;
    TS_Dist_Req=TS_Dist_Init;
    TS_SignName_Value_Req=TS_SignName_Value_Init;
    SPL_End_Req=false;
    SPL_EndDist_Req=single(0);
    SPL_Constancy_Req=uint8(0);
  state OFF
    TSRSts=uint8(0);
    SPL_noSupp_EnableReq=false;
    SPL_noSupp_Dist_Req=single(0);
    SPL_noSupp_Value_Req=uint8(0);
    SPL_whSupp_EnableReq=false;
    SPL_whSupp_Dist_Req=single(0);
    SPL_whSupp_Value_Req=uint8(0);
    SPL_SuppName_Value_Req=uint8(0);
    TS_EnableReq=false;
    TS_Dist_Req=single(0);
    TS_SignName_Value_Req=uint8(0);
    SPL_End_Req=false;
    SPL_EndDist_Req=single(0);
    SPL_Constancy_Req=uint8(0);
  state ERROR
    TSRSts=uint8(4);
    SPL_noSupp_EnableReq=false;
    SPL_noSupp_Dist_Req=single(0);
    SPL_noSupp_Value_Req=uint8(0);
    SPL_whSupp_EnableReq=false;
    SPL_whSupp_Dist_Req=single(0);
    SPL_whSupp_Value_Req=uint8(0);
    SPL_SuppName_Value_Req=uint8(0);
    TS_EnableReq=false;
    TS_Dist_Req=single(0);
    TS_SignName_Value_Req=uint8(0);
    SPL_End_Req=false;
    SPL_EndDist_Req=single(0);
    SPL_Constancy_Req=uint8(0);
  state ON
    TSRSts=FUSSts;
    SPL_noSupp_EnableReq=SPL_noSupp_EnableReq_Rt;
    SPL_noSupp_Dist_Req=SPL_noSupp_Dist_Rt;
    SPL_noSupp_Value_Req=SPL_noSupp_Value_Rt;
    SPL_whSupp_EnableReq=SPL_whSupp_EnableReq_Rt;
    SPL_whSupp_Dist_Req=SPL_whSupp_Dist_Rt;
    SPL_whSupp_Value_Req=SPL_whSupp_Value_Rt;
    SPL_SuppName_Value_Req=SPL_SuppName_Value_Rt;
    TS_EnableReq=TS_EnableReq_Rt;
    TS_Dist_Req=TS_Dist_Rt;
    TS_SignName_Value_Req=TS_SignName_Value_Rt;
    SPL_End_Req=SPL_End_Rt;
    SPL_EndDist_Req=SPL_EndDist_Rt;
    SPL_Constancy_Req=SPL_Constancy_Rt;
  (default) -> Start
  Start -> (junction 170) : [VehConfigTSR==1&&TSR_error~=3]
  (junction 170) -> (junction 171) [order 1] : [SPL_noSupp_Value_Init~=0]
  (junction 170) -> (junction 172) [order 2] : {SPL_noSupp_EnableReq=false;}
  (junction 171) -> (junction 172) : {SPL_noSupp_EnableReq=true;}
  (junction 172) -> (junction 180)
  (junction 180) -> (junction 179) [order 1] : [SPL_whSupp_Value_Init~=0]
  (junction 180) -> (junction 175) [order 2] : {SPL_whSupp_EnableReq=false;}
  (junction 179) -> (junction 175) : {SPL_whSupp_EnableReq=true;}
  (junction 175) -> (junction 212)
  (junction 212) -> (junction 213) [order 1] : [TS_SignName_Value_Init~=0]
  (junction 212) -> (junction 214) [order 2] : {TS_EnableReq=false;}
  (junction 213) -> (junction 214) : {TS_EnableReq=true;}
  (junction 214) -> INIT
  INIT -> OFF [order 3] : [TSR_error==3]
  INIT -> ERROR [order 2] : [TSR_error==1]
  INIT -> ON [order 1] : [TSR_error~=1&&TSR_error~=3]
  ERROR -> OFF [order 2] : [TSR_error==3]
  OFF -> ERROR [order 2] : [TSR_error==1]
  ERROR -> ON [order 1] : [TSR_error~=1&&...
      | TSR_error~=3]
  ON -> ERROR [order 2] : [TSR_error==1]
  OFF -> ON [order 1] : [TSR_error~=3&&TSR_error~=1]
  ON -> OFF [order 1] : [TSR_error==3]
  data: VehConfigTSR input uint8; TSR_error input uint8; FUSSts input uint8; TSRSts output uint8; SPL_noSupp_Value_Req output uint8; SPL_noSupp_Value_Init input uint8; SPL_noSupp_Dist_Init input single; SPL_whSupp_Value_Init input uint8; SPL_SuppName_Value_Init input uint8; SPL_whSupp_Dist_Init input single; TS_SignName_Value_Init input uint8; TS_Dist_Init input single; SPL_noSupp_EnableReq_Rt input boolean; SPL_noSupp_Dist_Req output single; SPL_whSupp_Value_Req output uint8; SPL_SuppName_Value_Req output uint8; SPL_whSupp_Dist_Req output single; TS_SignName_Value_Req output uint8; TS_Dist_Req output single; SPL_noSupp_Dist_Rt input single; SPL_noSupp_Value_Rt input uint8; SPL_whSupp_EnableReq_Rt input boolean; SPL_whSupp_Dist_Rt input single; SPL_whSupp_Value_Rt input uint8; SPL_SuppName_Value_Rt input uint8; SPL_End_Rt input boolean; SPL_EndDist_Rt input single; SPL_Constancy_Rt input uint8; TS_EnableReq_Rt input boolean; TS_Dist_Rt input single; TS_SignName_Value_Rt input uint8; SPL_noSupp_EnableReq output boolean; SPL_whSupp_EnableReq output boolean; TS_EnableReq output boolean; SPL_End_Req output boolean; SPL_EndDist_Req output single; SPL_Constancy_Req output uint8

== matlab function PvtSubSys_VSM_ALL/Subsystem/StateManage/EDR_HWAExit/MATLAB Function1 ==
  data: HWAExit_b input; y output boolean; CounterK1 input; Counter output
function [y, Counter] = fcn(HWAExit_b,CounterK1)
Counter = CounterK1;
if HWAExit_b==1
    Counter = 4;
end

if Counter>0
    Counter = Counter-1;    
    y = true;
else
    y = false;
    
end

== matlab function PvtSubSys_VSM_ALL/Subsystem/StateManage/EDR_HWAExit/MATLAB Function2 ==
  data: HWAExit_b input; y output boolean; CounterK1 input; Counter output
function [y, Counter] = fcn(HWAExit_b,CounterK1)
Counter = CounterK1;
if HWAExit_b==1
    Counter = 4;
end

if Counter>0
    Counter = Counter-1;    
    y = true;
else
    y = false;
    
end

== matlab function PvtSubSys_VSM_ALL/Subsystem/StateManage/EDR_HWAExit/MATLAB Function3 ==
  data: HWAExit_b input; y output boolean; CounterK1 input; Counter output
function [y, Counter] = fcn(HWAExit_b,CounterK1)
Counter = CounterK1;
if HWAExit_b==1
    Counter = 4;
end

if Counter>0
    Counter = Counter-1;    
    y = true;
else
    y = false;
    
end

== stateflow chart PvtSubSys_VSM_ALL/Subsystem/StateManage/Enlong2s1/Chart ==
  state NO
    en:
    SW = false;
  state YES
    en:
    SW = true;
  (default) -> NO
  NO -> YES : [state==true&&vehspd>P_VSM_SOSSpd_SW]
  YES -> NO : [ACCSOS == 1]
  data: P_VSM_SOSSpd_SW input; vehspd input; state input; SW output; ACCSOS input

== matlab function PvtSubSys_VSM_ALL/Subsystem/StateManage/Enlong2s1/MATLAB Function ==
  data: CntK1 input uint16; Cnt output uint16; X input; Num input
function Cnt= TextCount(CntK1,X,Num)

if X==true
    Cnt = Num;
else
     Cnt = max(CntK1-uint16(1),uint16(0));
end

== matlab function PvtSubSys_VSM_ALL/Subsystem/StateManage/LSS/LCK_LKA_LDW_ELKStateMachine3/LSSHMI/LSMC_Signal ==
  data: LCKState input; LDWState input; ELKState input; LKAState input; HandsOffWarnLevel input; Signal_HandsOffWarn output; ability input; LaneAvaliability output; TJASts input; LCK_TJASts input
function [Signal_HandsOffWarn,LaneAvaliability] = fcn(LCKState,LDWState, ELKState, LKAState,HandsOffWarnLevel,ability,TJASts,LCK_TJASts)

    LaneAvaliability=uint8(0);
if LCKState==1 || LDWState==1 || ELKState==1 || LKAState==1 || (LCK_TJASts==1 && TJASts==3) 
     LaneAvaliability=ability;
end
%% handoffwarn
Signal_HandsOffWarn = HandsOffWarnLevel;

== matlab function PvtSubSys_VSM_ALL/Subsystem/StateManage/LSS/LCK_LKA_LDW_ELKStateMachine3/LSSHMI/MATLAB Function ==
  data: LCK_Warn input; LKA_Warn input; Warn output; ELK_Warn input
function Warn = fcn(LCK_Warn, LKA_Warn, ELK_Warn)
Warn=0;
if ELK_Warn>0
    Warn=ELK_Warn;
elseif LKA_Warn>0
    Warn=LKA_Warn;
elseif LCK_Warn>0
    Warn=LCK_Warn;
end

== matlab function PvtSubSys_VSM_ALL/Subsystem/StateManage/LSS/LCK_LKA_LDW_ELKStateMachine3/LSSHMI/MATLAB Function2 ==
  data: LeftValid input; LaneAvailability output; RightValid input; LeftA0 input; RightA0 input; LaneWidth input
function LaneAvailability = fcn(LeftValid,RightValid,LeftA0,RightA0,LaneWidth)

 LaneAvailability=uint8(0);
 
if LeftValid==true && RightValid== true %% tow lane
    if LaneWidth>=5.5
        LaneAvailability=uint8(0);
        if LeftA0 < 2.75
            LaneAvailability=uint8(1);
        elseif RightA0> -2.75
            LaneAvailability=uint8(2);
        end
    elseif LaneWidth<5.5 && LaneWidth>2.5
         LaneAvailability=uint8(3);
    end
elseif LeftValid==true && RightValid==false %% left lane
    if LeftA0<2.75
        LaneAvailability=uint8(1);
    end
elseif LeftValid==false && RightValid==true %% right lane
    if RightA0>-2.75
         LaneAvailability=uint8(2);
    end
end

== matlab function PvtSubSys_VSM_ALL/Subsystem/StateManage/LSS/TargetLineSelect/Line ==
  data: HWAActive input; HWAsts input; y output; TJASts input; ELKSts input; LKASts input; LCKIESts input; ESS_Sts input; LCK_Sts input
function y = LineSelect(HWAActive,HWAsts, TJASts,ELKSts,LKASts,LCKIESts,ESS_Sts,LCK_Sts)
y=  7;
if HWAActive
    if LCK_Sts==LCK_STATE.LCK_Active
        y = 1;
    end
    if LCKIESts ==STATE.ACTIVE_LEFT && HWAsts~=5 && HWAsts~=6
        y= 5;
    elseif LCKIESts==STATE.ACTIVE_RIGHT && HWAsts~=5 && HWAsts~=6
        y= 6;
    end
elseif TJASts==3
    if LCK_Sts==LCK_STATE.LCK_Active
        y = 2;
    end
    if LCKIESts ==STATE.ACTIVE_LEFT && HWAsts~=5 && HWAsts~=6
        y= 5;
    elseif LCKIESts==STATE.ACTIVE_RIGHT && HWAsts~=5 && HWAsts~=6
        y= 6;
    end
elseif ELKSts==5 || ELKSts==7  %line    3:left; 4:right
    y = 3;
elseif  ELKSts==6 || ELKSts==8
    y = 3;
elseif ELKSts==3  % re                  5: left; 6: right
    y = 3;
elseif  ELKSts==4 
    y = 3;
elseif LKASts==STATE.ACTIVE_LEFT ||  LKASts==STATE.ACTIVE_RIGHT
    y =  4;
elseif ESS_Sts == 4 || ESS_Sts == 5
    y = 8;
end



end

== matlab function PvtSubSys_VSM_ALL/Subsystem/StateManage/MATLAB Function2 ==
  data: DriverSts input; DriverInloop_Monitor output
function DriverInloop_Monitor = fcn(DriverSts)

if (DriverSts == 0) || (DriverSts == 1)
    DriverInloop_Monitor = 0;
elseif (DriverSts == 2) || (DriverSts == 6)
    DriverInloop_Monitor = 1;
elseif (DriverSts == 3) || (DriverSts == 7)
    DriverInloop_Monitor = 2;
elseif (DriverSts == 4) || (DriverSts == 5) || (DriverSts == 8) || (DriverSts == 9)
    DriverInloop_Monitor = 3;
else
    DriverInloop_Monitor = 0;
end

== matlab function PvtSubSys_VSM_ALL/Subsystem/StateManage/MATLAB Function4 ==
  data: HWASts input; TJASts input; HWAAccControlSts output; DriverSts input
function HWAAccControlSts = fcn(HWASts,TJASts, DriverSts)

if HWASts == 9 || TJASts == 9
    HWAAccControlSts = 3;
elseif (HWASts == 5) || (HWASts == 6)
    HWAAccControlSts = 2;
elseif TJASts == 10
    HWAAccControlSts = 5;
elseif (DriverSts ~= 0) && (DriverSts ~= 1)
    HWAAccControlSts = 4;
else
    HWAAccControlSts = 0;
end
